simulink model "pulse_detector_v4_4"  (R2017b)
settings: Solver=FixedStepDiscrete  StartTime=0.0  StopTime=SimTime  RelTol=1e-3
undefined symbols (not defined in the file): CorrFilter, rowCorrFilter, RxSignal, threshold, WindowLen
libraries: dspsrcs4 x2, dsphdlfiltering x1, simulink x1, hdlsllib x1
settings Model: DataTypeOverride=Off  SimulationMode=accelerator  Creator=proso  LastModifiedBy=proso
settings DataIOCC: SaveOutput=off  SaveTime=off  ReturnWorkspaceOutputs=on
settings OptimizationCC: BlockReduction=off  ConditionallyExecuteInputs=off  DefaultParameterBehavior=Inlined
settings DebuggingCC: AlgebraicLoopMsg=error  SingleTaskRateTransMsg=error
settings HardwareCC: ProdBitPerPointer=32  ProdBitPerSizeT=32  ProdBitPerPtrDiffT=32  ProdLargestAtomicFloat=None  ProdIntDivRoundTo=Undefined  ProdEndianess=Unspecified  ProdWordSize=32  ProdHWDeviceType=ASIC/FPGA->ASIC/FPGA  TargetBitPerPointer=64  TargetBitPerSizeT=64  TargetBitPerPtrDiffT=64  TargetLongLongMode=on  TargetIntDivRoundTo=Zero  TargetEndianess=LittleEndian  TargetWordSize=64  TargetHWDeviceType=Custom Processor->MATLAB Host Computer  ProdEqTarget=off

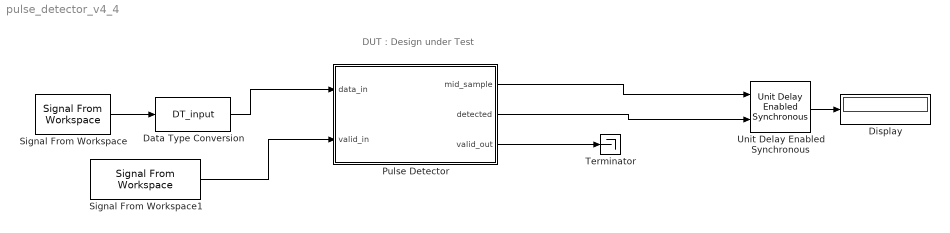
== system pulse_detector_v4_4 ==
  note: DUT : Design under Test
  Data Type Conversion : DataTypeConversion  OutDataTypeStr=DT_input
  Display : Display
  Pulse Detector : Subsystem
  Signal From Workspace : dspsrcs4/Signal From Workspace  X=RxSignal  Ts=1  nsamps=1  OutputAfterFinalValue=Setting to zero  ignoreOrWarnInputAndFrameLengths=off  OutputFrames=off
  Signal From Workspace1 : dspsrcs4/Signal From Workspace  X=true(size(RxSignal))  Ts=1  nsamps=1  OutputAfterFinalValue=Setting to zero  ignoreOrWarnInputAndFrameLengths=off  OutputFrames=off
  Terminator : Terminator
  Unit Delay Enabled Synchronous : hdlsllib/Discrete/Unit Delay Enabled Synchronous  InitialCondition=0.0  SampleTime=-1
      settings: SourceProductName=HDL Coder  SourceProductBaseCode=HD
  wires:
  Unit Delay Enabled Synchronous/1 -> Display/1
  Pulse Detector/1(mid_sample) -> Unit Delay Enabled Synchronous/1
  Pulse Detector/2(detected) -> Unit Delay Enabled Synchronous/2
  Signal From Workspace1/1 -> Pulse Detector/2(valid_in)
  Pulse Detector/3(valid_out) -> Terminator/1
  Signal From Workspace/1 -> Data Type Conversion/1
  Data Type Conversion/1 -> Pulse Detector/1(data_in)

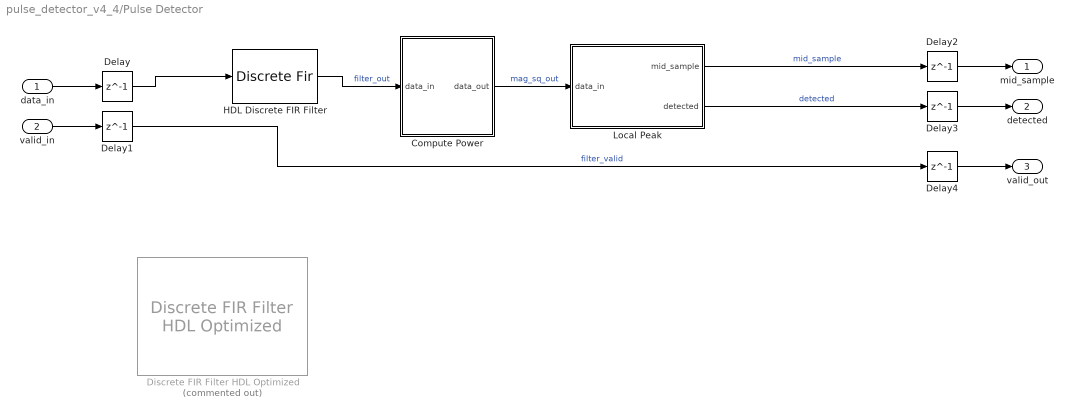
== system pulse_detector_v4_4/Pulse Detector ==
  data_in : Inport
  valid_in : Inport  Port=2
  Compute Power : Subsystem
  Delay{,1..4} (5 alike) : Delay  DelayLength=1
  Discrete FIR Filter HDL Optimized : dsphdlfiltering/Discrete FIR Filter HDL Optimized  Commented=on  Numerator=real(rowCorrFilter)  Sharing=off  SharingFactor=2  SimulateUsing=Code generation  roundingMode=Floor  overflowMode=off  CoefficientsDataTypeStr=DT_coeff  CoefficientsMin=[]  CoefficientsMax=[]  OutputDataTypeStr=Inherit: Same word length as input  OutputMin=[]  OutputMax=[]  ValidInPort=on  ReadyPort=off
      settings: SourceProductName=DSP System Toolbox  SourceProductBaseCode=DS
  HDL Discrete FIR Filter : DiscreteFir  FilterStructure=Direct form transposed  Coefficients=CorrFilter  CoefDataTypeStr=DT_coeff
  Local Peak : Subsystem
  mid_sample : Outport
  detected : Outport  Port=2
  valid_out : Outport  Port=3
  wires:
  HDL Discrete FIR Filter/1 -> Compute Power/1(data_in)  "filter_out"
  Compute Power/1(data_out) -> Local Peak/1(data_in)  "mag_sq_out"
  Local Peak/1(mid_sample) -> Delay2/1  "mid_sample"
  data_in/1 -> Delay/1
  Local Peak/2(detected) -> Delay3/1  "detected"
  valid_in/1 -> Delay1/1
  Delay1/1 -> Delay4/1  "filter_valid"
  Delay/1 -> HDL Discrete FIR Filter/1
  Delay2/1 -> mid_sample/1
  Delay3/1 -> detected/1
  Delay4/1 -> valid_out/1

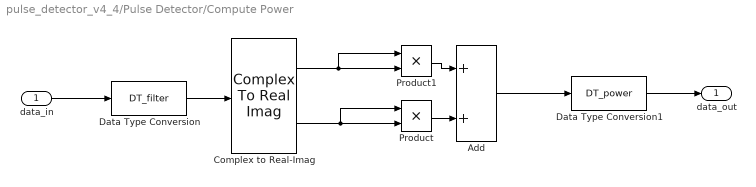
== system pulse_detector_v4_4/Pulse Detector/Compute Power ==
  data_in : Inport
  Add : Sum
  Complex to Real-Imag : ComplexToRealImag
  Data Type Conversion : DataTypeConversion  OutDataTypeStr=DT_filter
  Data Type Conversion1 : DataTypeConversion  OutDataTypeStr=DT_power
  Product : Product
  Product1 : Product
  data_out : Outport
  wires:
  Product1/1 -> Add/1
  data_in/1 -> Data Type Conversion/1
  Complex to Real-Imag/1 -> Product1/1, Product1/2
  Add/1 -> Data Type Conversion1/1
  Product/1 -> Add/2
  Complex to Real-Imag/2 -> Product/1, Product/2
  Data Type Conversion/1 -> Complex to Real-Imag/1
  Data Type Conversion1/1 -> data_out/1

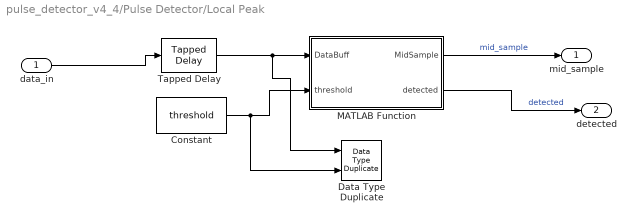
== system pulse_detector_v4_4/Pulse Detector/Local Peak ==
  data_in : Inport
  Constant : Constant  Value=threshold  OutDataTypeStr=Inherit: Inherit via back propagation  SampleTime=-1
  Data Type Duplicate : DataTypeDuplicate
  MATLAB Function : MATLAB Function  TreatAsAtomicUnit=on
  Tapped Delay : simulink/Discrete/Tapped Delay  vinit=0.0  samptime=-1  NumDelays=WindowLen  DelayOrder=Oldest  includeCurrent=off
  mid_sample : Outport
  detected : Outport  Port=2
  wires:
  MATLAB Function/1(MidSample) -> mid_sample/1  "mid_sample"
  data_in/1 -> Tapped Delay/1
  MATLAB Function/2(detected) -> detected/1  "detected"
  Tapped Delay/1 -> Data Type Duplicate/1, MATLAB Function/1(DataBuff)
  Constant/1 -> Data Type Duplicate/2, MATLAB Function/2(threshold)

== matlab function pulse_detector_v4_4/Pulse Detector/Local Peak/MATLAB Function ==
  settings: fimath=fimath('RoundingMethod', 'Floor','OverflowAction', 'Wrap','ProductMode', 'FullPrecision', 'SumMode', 'FullPrecision')
  data: MidSample output; DataBuff input; threshold input; detected output; WindowLen parameter
function [MidSample,detected] = fcn(DataBuff,threshold, WindowLen)
   
MidIdx = ceil(WindowLen/2);
% Sliding window operation

% Compare each value in the window to the middle sample via subtraction
MidSample = DataBuff(MidIdx);
CompareOut = DataBuff - MidSample; % this is a vector

% if all values in the result are negative and the middle sample is
% greater than a threshold, it is a local max
if all(CompareOut <= 0) && (MidSample > threshold)
    detected = true;
else 
    detected = false;
end
